simulink model "flightController"  (R2021a)
settings: Solver=ode3  StartTime=0  StopTime=10  FixedStep=Ts  RelTol=1e-3  EnableMultiTasking=on
undefined symbols (not defined in the file): Controller, ControlvsRed, D_ROLL, delays, DiscIntNeverNeededParam, g, I_ROLL, norm_act, Normalization, P_Pitch, P_ROLL, P_Roll, P_Yaw, P_z, PR_Start, save_time, sts_cnames, time_DisYaw, time_stepsX, time_stepsY, time_stepsZ, Ts, Vehicle, x0, x0_f
libraries: deeplib x5
(part 4 of 4)

== system flightController/Variant Subsystem/ANN_Feedback/Subsystem1/Subsystem12/Subsystem3 ==
  <Z> : Inport
  Constant : Constant  Value=Normalization(3,2)
  Gain : Gain  Gain=1/(Normalization(3,1)-Normalization(3,2))
  Sum : Sum  Inputs=|+-
  Z : Outport
  wires:
  <Z>/1 -> Sum/1
  Gain/1 -> Z/1
  Sum/1 -> Gain/1
  Constant/1 -> Sum/2

== system flightController/Variant Subsystem/ANN_Feedback/Subsystem1/Subsystem12/Subsystem4 ==
  <dz> : Inport
  Constant : Constant  Value=Normalization(6,2)
  Gain : Gain  Gain=1/(Normalization(6,1)-Normalization(6,2))
  Sum : Sum  Inputs=|+-
  Dz : Outport
  wires:
  Sum/1 -> Gain/1
  <dz>/1 -> Sum/1
  Constant/1 -> Sum/2
  Gain/1 -> Dz/1

== system flightController/Variant Subsystem/ANN_Feedback/Subsystem1/Subsystem12/Subsystem6 ==
  <Acel_z> : Inport
  Constant : Constant  Value=Normalization(30,2)
  Gain : Gain  Gain=1/(Normalization(30,1)-Normalization(30,2))
  Sum : Sum  Inputs=|+-
  Acceleracion Z : Outport
  wires:
  Sum/1 -> Gain/1
  <Acel_z>/1 -> Sum/1
  Constant/1 -> Sum/2
  Gain/1 -> Acceleracion Z/1

== system flightController/Variant Subsystem/ANN_Feedback/Subsystem1/Subsystem12/Subsystem7 ==
  <Ac_Dz> : Inport
  Constant : Constant  Value=Normalization(18,2)
  Gain : Gain  Gain=1/(Normalization(18,1)-Normalization(18,2))
  Sum : Sum  Inputs=|+-
  Ac_Dz : Outport
  wires:
  Gain/1 -> Ac_Dz/1
  Constant/1 -> Sum/2
  Sum/1 -> Gain/1
  <Ac_Dz>/1 -> Sum/1

== system flightController/Variant Subsystem/ANN_Feedback/Subsystem1/Subsystem12/Subsystem8 ==
  <Pressure Altitud> : Inport
  Constant : Constant  Value=Normalization(26,2)
  Gain : Gain  Gain=1/(Normalization(26,1)-Normalization(26,2))
  Sum : Sum  Inputs=|+-
  Pressure Altitud : Outport
  wires:
  Gain/1 -> Pressure Altitud/1
  Constant/1 -> Sum/2
  Sum/1 -> Gain/1
  <Pressure Altitud>/1 -> Sum/1

== system flightController/Variant Subsystem/ANN_Feedback/Subsystem1/Subsystem12/Subsystem9 ==
  <Sonar Altitud> : Inport
  Constant : Constant  Value=Normalization(22,2)
  Gain : Gain  Gain=1/(Normalization(22,1)-Normalization(22,2))
  Sum : Sum  Inputs=|+-
  Sonar Altitud : Outport
  wires:
  Gain/1 -> Sonar Altitud/1
  Constant/1 -> Sum/2
  Sum/1 -> Gain/1
  <Sonar Altitud>/1 -> Sum/1

== system flightController/Variant Subsystem/ANN_Feedback/Subsystem1/Subsystem13/Subsystem1 ==
  <Z> : Inport
  Constant : Constant  Value=Normalization(2,2)
  Gain : Gain  Gain=1/(Normalization(2,1)-Normalization(2,2))
  Sum : Sum  Inputs=|+-
  Z : Outport
  wires:
  Constant/1 -> Sum/2
  Sum/1 -> Gain/1
  Gain/1 -> Z/1
  <Z>/1 -> Sum/1

== system flightController/Variant Subsystem/ANN_Feedback/Subsystem1/Subsystem13/Subsystem10 ==
  <Z> : Inport
  Constant : Constant  Value=Normalization(11,2)
  Gain : Gain  Gain=1/(Normalization(11,1)-Normalization(11,2))
  Sum : Sum  Inputs=|+-
  Z : Outport
  wires:
  Constant/1 -> Sum/2
  Sum/1 -> Gain/1
  Gain/1 -> Z/1
  <Z>/1 -> Sum/1

== system flightController/Variant Subsystem/ANN_Feedback/Subsystem1/Subsystem13/Subsystem11 ==
  In1 : Inport
  Constant1 : Constant  Value=Ts
  Delay1 : Delay  DelayLength=1  InitialCondition=0
  Divide1 : Product  Inputs=*/
  Sum1 : Sum  Inputs=|+-
  <Acel_Z> : Outport
  wires:
  Divide1/1 -> <Acel_Z>/1
  Delay1/1 -> Sum1/2
  Sum1/1 -> Divide1/1
  Constant1/1 -> Divide1/2
  In1/1 -> Sum1/1, Delay1/1

== system flightController/Variant Subsystem/ANN_Feedback/Subsystem1/Subsystem13/Subsystem12 ==
  <Acel_z> : Inport
  Constant : Constant  Value=Normalization(24,2)
  Gain : Gain  Gain=1/(Normalization(24,1)-Normalization(24,2))
  Sum : Sum  Inputs=|+-
  Acceleracion Z : Outport
  wires:
  Sum/1 -> Gain/1
  <Acel_z>/1 -> Sum/1
  Constant/1 -> Sum/2
  Gain/1 -> Acceleracion Z/1

== system flightController/Variant Subsystem/ANN_Feedback/Subsystem1/Subsystem13/Subsystem13 ==
  In1 : Inport
  Constant1 : Constant  Value=Ts
  Delay1 : Delay  DelayLength=1  InitialCondition=0
  Divide1 : Product  Inputs=*/
  Sum1 : Sum  Inputs=|+-
  <Acel_Z> : Outport
  wires:
  Divide1/1 -> <Acel_Z>/1
  Delay1/1 -> Sum1/2
  Sum1/1 -> Divide1/1
  Constant1/1 -> Divide1/2
  In1/1 -> Sum1/1, Delay1/1

== system flightController/Variant Subsystem/ANN_Feedback/Subsystem1/Subsystem13/Subsystem14 ==
  <Acel_z> : Inport
  Constant : Constant  Value=Normalization(25,2)
  Gain : Gain  Gain=1/(Normalization(25,1)-Normalization(25,2))
  Sum : Sum  Inputs=|+-
  Acceleracion Z : Outport
  wires:
  Sum/1 -> Gain/1
  <Acel_z>/1 -> Sum/1
  Constant/1 -> Sum/2
  Gain/1 -> Acceleracion Z/1

== system flightController/Variant Subsystem/ANN_Feedback/Subsystem1/Subsystem13/Subsystem15 ==
  In1 : Inport
  Constant1 : Constant  Value=Ts
  Delay1 : Delay  DelayLength=1  InitialCondition=0
  Divide1 : Product  Inputs=*/
  Sum1 : Sum  Inputs=|+-
  <Acel_Z> : Outport
  wires:
  Divide1/1 -> <Acel_Z>/1
  Delay1/1 -> Sum1/2
  Sum1/1 -> Divide1/1
  Constant1/1 -> Divide1/2
  In1/1 -> Sum1/1, Delay1/1

== system flightController/Variant Subsystem/ANN_Feedback/Subsystem1/Subsystem13/Subsystem16 ==
  <Acel_z> : Inport
  Constant : Constant  Value=Normalization(26,2)
  Gain : Gain  Gain=1/(Normalization(26,1)-Normalization(26,2))
  Sum : Sum  Inputs=|+-
  Acceleracion Z : Outport
  wires:
  Sum/1 -> Gain/1
  <Acel_z>/1 -> Sum/1
  Constant/1 -> Sum/2
  Gain/1 -> Acceleracion Z/1

== system flightController/Variant Subsystem/ANN_Feedback/Subsystem1/Subsystem13/Subsystem17 ==
  <Y> : Inport
  Constant : Constant  Value=Normalization(2,2)
  Gain : Gain  Gain=1/(Normalization(2,1)-Normalization(2,2))
  Sum : Sum  Inputs=|+-
  Y : Outport
  wires:
  Constant/1 -> Sum/2
  Sum/1 -> Gain/1
  Gain/1 -> Y/1
  <Y>/1 -> Sum/1

== system flightController/Variant Subsystem/ANN_Feedback/Subsystem1/Subsystem13/Subsystem18 ==
  <X> : Inport
  Constant : Constant  Value=Normalization(1,2)
  Gain : Gain  Gain=1/(Normalization(1,1)-Normalization(1,2))
  Sum : Sum  Inputs=|+-
  X : Outport
  wires:
  <X>/1 -> Sum/1
  Gain/1 -> X/1
  Sum/1 -> Gain/1
  Constant/1 -> Sum/2

== system flightController/Variant Subsystem/ANN_Feedback/Subsystem1/Subsystem13/Subsystem19 ==
  <dy> : Inport
  Constant : Constant  Value=Normalization(7,2)
  Gain : Gain  Gain=1/(Normalization(7,1)-Normalization(7,2))
  Sum : Sum  Inputs=|+-
  Dy : Outport
  wires:
  Sum/1 -> Gain/1
  <dy>/1 -> Sum/1
  Constant/1 -> Sum/2
  Gain/1 -> Dy/1

== system flightController/Variant Subsystem/ANN_Feedback/Subsystem1/Subsystem13/Subsystem2 ==
  <Z> : Inport
  Constant : Constant  Value=Normalization(4,2)
  Gain : Gain  Gain=1/(Normalization(4,1)-Normalization(4,2))
  Sum : Sum  Inputs=|+-
  Z : Outport
  wires:
  Constant/1 -> Sum/2
  Sum/1 -> Gain/1
  Gain/1 -> Z/1
  <Z>/1 -> Sum/1

== system flightController/Variant Subsystem/ANN_Feedback/Subsystem1/Subsystem13/Subsystem20 ==
  <dx> : Inport
  Constant : Constant  Value=Normalization(6,2)
  Gain : Gain  Gain=1/(Normalization(6,1)-Normalization(6,2))
  Sum : Sum  Inputs=|+-
  Dx : Outport
  wires:
  Gain/1 -> Dx/1
  Constant/1 -> Sum/2
  <dx>/1 -> Sum/1
  Sum/1 -> Gain/1

== system flightController/Variant Subsystem/ANN_Feedback/Subsystem1/Subsystem13/Subsystem21 ==
  In1 : Inport
  Constant1 : Constant  Value=Ts
  Delay1 : Delay  DelayLength=1  InitialCondition=0
  Divide1 : Product  Inputs=*/
  Sum1 : Sum  Inputs=|+-
  <Acel_Y> : Outport
  wires:
  Divide1/1 -> <Acel_Y>/1
  Delay1/1 -> Sum1/2
  Sum1/1 -> Divide1/1
  Constant1/1 -> Divide1/2
  In1/1 -> Sum1/1, Delay1/1

== system flightController/Variant Subsystem/ANN_Feedback/Subsystem1/Subsystem13/Subsystem22 ==
  <Acel_y> : Inport
  Constant : Constant  Value=Normalization(21,2)
  Gain : Gain  Gain=1/(Normalization(21,1)-Normalization(21,2))
  Sum : Sum  Inputs=|+-
  Acceleracion Y : Outport
  wires:
  Sum/1 -> Gain/1
  <Acel_y>/1 -> Sum/1
  Constant/1 -> Sum/2
  Gain/1 -> Acceleracion Y/1

== system flightController/Variant Subsystem/ANN_Feedback/Subsystem1/Subsystem13/Subsystem23 ==
  In1 : Inport
  Constant1 : Constant  Value=Ts
  Delay1 : Delay  DelayLength=1  InitialCondition=0
  Divide1 : Product  Inputs=*/
  Sum1 : Sum  Inputs=|+-
  <Acel_X> : Outport
  wires:
  In1/1 -> Delay1/1, Sum1/1
  Constant1/1 -> Divide1/2
  Sum1/1 -> Divide1/1
  Delay1/1 -> Sum1/2
  Divide1/1 -> <Acel_X>/1

== system flightController/Variant Subsystem/ANN_Feedback/Subsystem1/Subsystem13/Subsystem24 ==
  <Acel_x> : Inport
  Constant : Constant  Value=Normalization(20,2)
  Gain : Gain  Gain=1/(Normalization(20,1)-Normalization(20,2))
  Sum : Sum  Inputs=|+-
  Acceleracion X : Outport
  wires:
  Gain/1 -> Acceleracion X/1
  Constant/1 -> Sum/2
  <Acel_x>/1 -> Sum/1
  Sum/1 -> Gain/1

== system flightController/Variant Subsystem/ANN_Feedback/Subsystem1/Subsystem13/Subsystem3 ==
  <Z> : Inport
  Constant : Constant  Value=Normalization(3,2)
  Gain : Gain  Gain=1/(Normalization(3,1)-Normalization(3,2))
  Sum : Sum  Inputs=|+-
  Z : Outport
  wires:
  Constant/1 -> Sum/2
  Sum/1 -> Gain/1
  Gain/1 -> Z/1
  <Z>/1 -> Sum/1

== system flightController/Variant Subsystem/ANN_Feedback/Subsystem1/Subsystem13/Subsystem4 ==
  <dz> : Inport
  Constant : Constant  Value=Normalization(8,2)
  Gain : Gain  Gain=1/(Normalization(8,1)-Normalization(8,2))
  Sum : Sum  Inputs=|+-
  Dz : Outport
  wires:
  Gain/1 -> Dz/1
  Constant/1 -> Sum/2
  <dz>/1 -> Sum/1
  Sum/1 -> Gain/1

== system flightController/Variant Subsystem/ANN_Feedback/Subsystem1/Subsystem13/Subsystem5 ==
  In1 : Inport
  Constant1 : Constant  Value=Ts
  Delay1 : Delay  DelayLength=1  InitialCondition=0
  Divide1 : Product  Inputs=*/
  Sum1 : Sum  Inputs=|+-
  <Acel_Z> : Outport
  wires:
  In1/1 -> Delay1/1, Sum1/1
  Constant1/1 -> Divide1/2
  Sum1/1 -> Divide1/1
  Delay1/1 -> Sum1/2
  Divide1/1 -> <Acel_Z>/1

== system flightController/Variant Subsystem/ANN_Feedback/Subsystem1/Subsystem13/Subsystem6 ==
  <Acel_z> : Inport
  Constant : Constant  Value=Normalization(22,2)
  Gain : Gain  Gain=1/(Normalization(22,1)-Normalization(22,2))
  Sum : Sum  Inputs=|+-
  Acceleracion Z : Outport
  wires:
  Gain/1 -> Acceleracion Z/1
  Constant/1 -> Sum/2
  <Acel_z>/1 -> Sum/1
  Sum/1 -> Gain/1

== system flightController/Variant Subsystem/ANN_Feedback/Subsystem1/Subsystem13/Subsystem7 ==
  <Z> : Inport
  Constant : Constant  Value=Normalization(5,2)
  Gain : Gain  Gain=1/(Normalization(5,1)-Normalization(5,2))
  Sum : Sum  Inputs=|+-
  Z : Outport
  wires:
  Constant/1 -> Sum/2
  Sum/1 -> Gain/1
  Gain/1 -> Z/1
  <Z>/1 -> Sum/1

== system flightController/Variant Subsystem/ANN_Feedback/Subsystem1/Subsystem13/Subsystem8 ==
  <dz> : Inport
  Constant : Constant  Value=Normalization(9,2)
  Gain : Gain  Gain=1/(Normalization(9,1)-Normalization(9,2))
  Sum : Sum  Inputs=|+-
  Dz : Outport
  wires:
  Sum/1 -> Gain/1
  <dz>/1 -> Sum/1
  Constant/1 -> Sum/2
  Gain/1 -> Dz/1

== system flightController/Variant Subsystem/ANN_Feedback/Subsystem1/Subsystem13/Subsystem9 ==
  <Z> : Inport
  Constant : Constant  Value=Normalization(10,2)
  Gain : Gain  Gain=1/(Normalization(10,1)-Normalization(10,2))
  Sum : Sum  Inputs=|+-
  Z : Outport
  wires:
  Constant/1 -> Sum/2
  Sum/1 -> Gain/1
  Gain/1 -> Z/1
  <Z>/1 -> Sum/1

== system flightController/Variant Subsystem/ANN_Feedback/Subsystem1/Subsystem3/Subsystem ==
  <Z_r> : Inport
  Constant : Constant  Value=Normalization(14,2)
  Gain : Gain  Gain=1/(Normalization(14,1)-Normalization(14,2))
  Sum : Sum  Inputs=|+-
  Z_r : Outport
  wires:
  <Z_r>/1 -> Sum/1
  Sum/1 -> Gain/1
  Constant/1 -> Sum/2
  Gain/1 -> Z_r/1

== system flightController/Variant Subsystem/ANN_Feedback/Subsystem1/Subsystem3/Subsystem1 ==
  In1 : Inport
  Constant1 : Constant  Value=Ts
  Delay1 : Delay  DelayLength=1  InitialCondition=0
  Divide1 : Product  Inputs=*/
  Sum1 : Sum  Inputs=|+-
  Out1 : Outport
  wires:
  In1/1 -> Delay1/1, Sum1/1
  Constant1/1 -> Divide1/2
  Sum1/1 -> Divide1/1
  Delay1/1 -> Sum1/2
  Divide1/1 -> Out1/1

== system flightController/Variant Subsystem/ANN_Feedback/Subsystem1/Subsystem3/Subsystem10 ==
  <X_r> : Inport
  Constant : Constant  Value=Normalization(12,2)
  Gain : Gain  Gain=1/(Normalization(12,1)-Normalization(12,2))
  Sum : Sum  Inputs=|+-
  X_r : Outport
  wires:
  <X_r>/1 -> Sum/1
  Sum/1 -> Gain/1
  Constant/1 -> Sum/2
  Gain/1 -> X_r/1

== system flightController/Variant Subsystem/ANN_Feedback/Subsystem1/Subsystem3/Subsystem11 ==
  <Dy_r> : Inport
  Constant : Constant  Value=Normalization(18,2)
  Gain : Gain  Gain=1/(Normalization(18,1)-Normalization(18,2))
  Sum : Sum  Inputs=|+-
  Dy_r : Outport
  wires:
  Gain/1 -> Dy_r/1
  Constant/1 -> Sum/2
  Sum/1 -> Gain/1
  <Dy_r>/1 -> Sum/1

== system flightController/Variant Subsystem/ANN_Feedback/Subsystem1/Subsystem3/Subsystem12 ==
  <Dx_r> : Inport
  Constant : Constant  Value=Normalization(17,2)
  Gain : Gain  Gain=1/(Normalization(17,1)-Normalization(17,2))
  Sum : Sum  Inputs=|+-
  Dx_r : Outport
  wires:
  <Dx_r>/1 -> Sum/1
  Sum/1 -> Gain/1
  Constant/1 -> Sum/2
  Gain/1 -> Dx_r/1

== system flightController/Variant Subsystem/ANN_Feedback/Subsystem1/Subsystem3/Subsystem2 ==
  <Dz_r> : Inport
  Constant : Constant  Value=Normalization(19,2)
  Gain : Gain  Gain=1/(Normalization(19,1)-Normalization(19,2))
  Sum : Sum  Inputs=|+-
  Dz_r : Outport
  wires:
  <Dz_r>/1 -> Sum/1
  Sum/1 -> Gain/1
  Constant/1 -> Sum/2
  Gain/1 -> Dz_r/1

== system flightController/Variant Subsystem/ANN_Feedback/Subsystem1/Subsystem3/Subsystem3 ==
  <Z_r> : Inport
  Constant : Constant  Value=0
  Constant1 : Constant  Commented=on  Value=Normalization(5,2)
  Gain : Gain  Commented=on  Gain=1/(Normalization(10,1)-Normalization(10,2))
  Gain1 : Gain
  Sum : Sum  Inputs=|+-
  Z_r : Outport
  wires:
  <Z_r>/1 -> Sum/1
  Constant/1 -> Sum/2
  Sum/1 -> Gain1/1
  Gain1/1 -> Z_r/1

== system flightController/Variant Subsystem/ANN_Feedback/Subsystem1/Subsystem3/Subsystem4 ==
  <Z_r> : Inport
  Constant : Constant  Value=Normalization(15,2)
  Gain : Gain  Commented=on  Gain=1/(Normalization(11,1)-Normalization(11,2))
  Sum : Sum  Inputs=|+-
  Z_r : Outport
  wires:
  <Z_r>/1 -> Sum/1
  Constant/1 -> Sum/2
  Sum/1 -> Z_r/1

== system flightController/Variant Subsystem/ANN_Feedback/Subsystem1/Subsystem3/Subsystem5 ==
  <Z_r> : Inport
  Constant : Constant  Value=Normalization(16,2)
  Gain : Gain  Commented=on  Gain=1/(Normalization(7,1)-Normalization(7,2))
  Gain1 : Gain
  Sum : Sum  Inputs=|+-
  Z_r : Outport
  wires:
  <Z_r>/1 -> Sum/1
  Constant/1 -> Sum/2
  Sum/1 -> Gain1/1
  Gain1/1 -> Z_r/1

== system flightController/Variant Subsystem/ANN_Feedback/Subsystem1/Subsystem3/Subsystem6 ==
  <Dz_r> : Inport
  Constant : Constant  Value=Normalization(14,2)
  Gain : Gain  Commented=on  Gain=1/(Normalization(14,1)-Normalization(14,2))
  Gain1 : Gain
  Sum : Sum  Inputs=|+-
  Dz_r : Outport
  wires:
  <Dz_r>/1 -> Sum/1
  Constant/1 -> Sum/2
  Sum/1 -> Gain1/1
  Gain1/1 -> Dz_r/1

== system flightController/Variant Subsystem/ANN_Feedback/Subsystem1/Subsystem3/Subsystem7 ==
  <Dz_r> : Inport
  Constant : Constant  Value=Normalization(15,2)
  Gain : Gain  Gain=1/(Normalization(15,1)-Normalization(15,2))
  Sum : Sum  Inputs=|+-
  Dz_r : Outport
  wires:
  <Dz_r>/1 -> Sum/1
  Sum/1 -> Gain/1
  Constant/1 -> Sum/2
  Gain/1 -> Dz_r/1

== system flightController/Variant Subsystem/ANN_Feedback/Subsystem1/Subsystem3/Subsystem8 ==
  <Dz_r> : Inport
  Constant : Constant  Value=Normalization(16,2)
  Gain : Gain  Gain=1/(Normalization(16,1)-Normalization(16,2))
  Sum : Sum  Inputs=|+-
  Dz_r : Outport
  wires:
  <Dz_r>/1 -> Sum/1
  Sum/1 -> Gain/1
  Constant/1 -> Sum/2
  Gain/1 -> Dz_r/1

== system flightController/Variant Subsystem/ANN_Feedback/Subsystem1/Subsystem3/Subsystem9 ==
  <Y_r> : Inport
  Constant : Constant  Value=Normalization(13,2)
  Gain : Gain  Gain=1/(Normalization(13,1)-Normalization(13,2))
  Sum : Sum  Inputs=|+-
  Y_r : Outport
  wires:
  Gain/1 -> Y_r/1
  Constant/1 -> Sum/2
  Sum/1 -> Gain/1
  <Y_r>/1 -> Sum/1

== matlab function flightController/Variant Subsystem/ANN_Feedback/Subsystem2/MATLAB Function ==
  data: out2 output; u input; y output; normalization input; Buffer input; Buffer output
function [out2,y,Buffer] = fcn(u, normalization, Buffer)

y=zeros(1,length(normalization(:,1)));

for i=1:length(normalization(:,1))
    %disp(normalization(:,3))
    if normalization(i,2)==normalization(i,1)
        y(1,i)=u(normalization(i,3));
    else
        y(1,i)=((u(normalization(i,3))-normalization(i,2))/(normalization(i,1)-normalization(i,2)));   
    end
    if y(1,i)>1 | y(1,i)<0
        disp("Fuera de los limites")
    end
    if y(1,i)==Inf
        disp("Infinito!!")
        disp(y(1,i))
    end
    if y(1,i)>1
        disp("Fuera de los limites")
    end
end

Buffer=circshift(Buffer,[0 1]);

Buffer(:,1)=y;
%disp("Size")
%disp()
size_Buffer=size(Buffer)
%flip(Buffer,2)
out2=reshape(Buffer,1,size_Buffer(1)*size_Buffer(2));

== matlab function flightController/Variant Subsystem/LSTM/Subsystem2/MATLAB Function ==
  data: u input; y output; normalization input; Buffer input; Buffer output
function [y,Buffer] = fcn(u, normalization, Buffer)

y=zeros(1,length(normalization(:,1)));

for i=1:length(normalization(:,1))
    %disp(normalization(:,3))
    if normalization(i,2)==normalization(i,1)
        y(1,i)=u(normalization(i,3));
    else
        y(1,i)=((u(normalization(i,3))-normalization(i,2))/(normalization(i,1)-normalization(i,2)));   
    end
    if y(1,i)>1 | y(1,i)<0
        disp("Fuera de los limites")
        disp(normalization(i,3))
    end
    if y(1,i)==Inf
        disp("Infinito!!")
        disp(y(1,i))
    end
    if y(1,i)>1
        disp("Fuera de los limites")
    end
end

Buffer=circshift(Buffer,[0 1]);

Buffer(:,1)=y;

== matlab function flightController/Variant Subsystem/LSTM/Subsystem3/MATLAB Function ==
  data: u input; y output; normalization input; Buffer input; Buffer output
function [y,Buffer] = fcn(u, normalization, Buffer)

y=zeros(1,length(normalization(:,1)));

for i=1:length(normalization(:,1))
    if normalization(i,2)==normalization(i,1)
        y(1,i)=u(normalization(i,3))
    else
        y(1,i)=((u(normalization(i,3))-normalization(i,2))/(normalization(i,1)-normalization(i,2)));   
    end
    if y(1,i)>1 | y(1,i)<0
        disp("Fuera de los limites")
    end
    if y(1,i)==Inf
        disp(y(1,i))
    end
end

Buffer=circshift(Buffer,[0 1]);
disp("OUT OF THE FEEDBACK")
disp(size(u(length(u)+1-(4*3):end)))
disp(size(y))
%Buffer=Buffer;
Buffer(:,1)=cat(2,y,u(length(u)+1-(4*3):end))
disp(size(Buffer(:,1)));

== matlab function flightController/Variant Subsystem/ANN/Subsystem2/MATLAB Function ==
  data: out2 output; u input; y output; normalization input; Buffer input; Buffer output
function [out2,y,Buffer] = fcn(u, normalization, Buffer)

y=zeros(1,length(normalization(:,1)));

for i=1:length(normalization(:,1))
    %disp(normalization(:,3))
    if normalization(i,2)==normalization(i,1)
        y(1,i)=u(normalization(i,3));
    else
        y(1,i)=((u(normalization(i,3))-normalization(i,2))/(normalization(i,1)-normalization(i,2)));   
    end
    if y(1,i)>1 | y(1,i)<0
        disp("Fuera de los limites")
    end
    if y(1,i)==Inf
        disp("Infinito!!")
        disp(y(1,i))
    end
    if y(1,i)>1
        disp("Fuera de los limites")
    end
end

Buffer=circshift(Buffer,[0 1]);

Buffer(:,1)=y;
%disp("Size")
%disp(size(Buffer))
%flip(Buffer,2)
size_Buffer=size(Buffer)
out2=reshape(Buffer,1,size_Buffer(1)*size_Buffer(2));;
